simulink model "Digital_Input_Block"  (R2021a)
settings: Solver=FixedStepDiscrete  StartTime=0.0  StopTime=inf  FixedStep=1e-3  RelTol=1e-3  EnableMultiTasking=on
libraries: simulink x9, arduinolib x9
settings Model: SILPILModeSetting=veronly  ExtModeTrigDuration=2  Creator=Admin  LastModifiedBy=Admin
settings OptimizationCC: EnhancedBackFolding=on  PassReuseOutputArgsAs=Individual arguments  ZeroExternalMemoryAtStartup=off  ZeroInternalMemoryAtStartup=off  MaxStackSize=64  OptimizeBlockOrder=speed  DifferentSizesBufferReuse=on  OptimizationCustomize=off  EfficientTunableParamExpr=on
settings DebuggingCC: ParameterTunabilityLossMsg=error
settings HardwareCC: ProdBitPerInt=16  ProdBitPerPointer=16  ProdBitPerSizeT=16  ProdBitPerPtrDiffT=16  ProdLargestAtomicFloat=None  ProdWordSize=8  ProdHWDeviceType=Atmel->AVR
settings SFSimCC: MATLABDynamicMemAlloc=off
settings RTWCC: SystemTargetFile=ert.tlc  HardwareBoard=Arduino Uno  TemplateMakefile=ert_default_tmf  Toolchain=Arduino AVR  BuildConfiguration=Faster Runs
settings CodeAppCC: ForceParamTrailComments=on  IgnoreCustomStorageClasses=off  OperatorAnnotations=on  SimulinkDataObjDesc=on  SFDataObjDesc=on  InsertBlockDesc=on
settings ERTTargetCC: SupportContinuousTime=on  SupportVariableSizeSignals=on  ExtModeStaticAllocSize=250

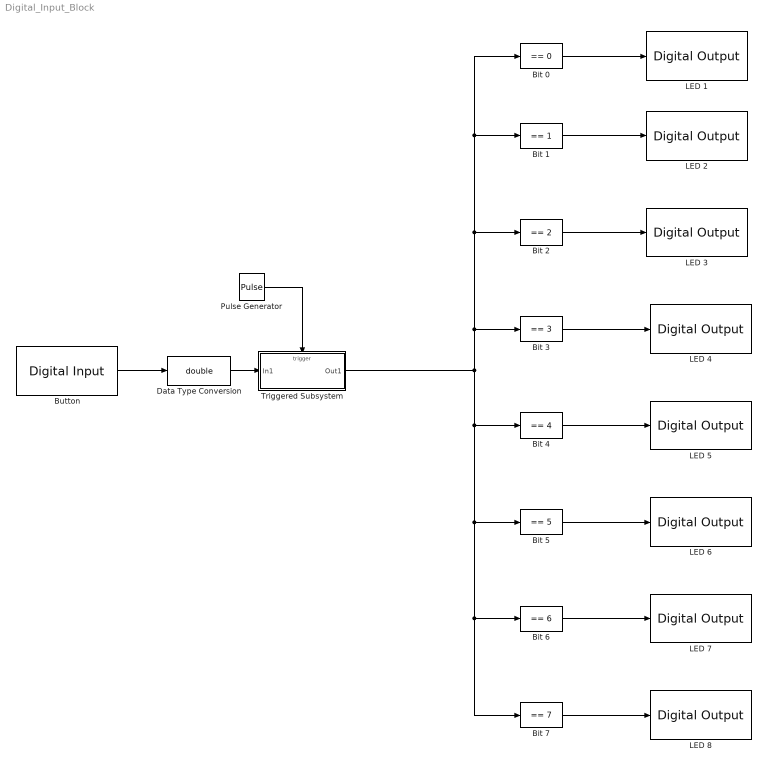
== system Digital_Input_Block ==
  Bit 0 : simulink/Logic and Bit Operations/Compare To Constant  relop===  const=0  OutDataTypeStr=boolean
  Bit 1 : simulink/Logic and Bit Operations/Compare To Constant  relop===  const=1  OutDataTypeStr=boolean
  Bit 2 : simulink/Logic and Bit Operations/Compare To Constant  relop===  const=2  OutDataTypeStr=boolean
  Bit 3 : simulink/Logic and Bit Operations/Compare To Constant  relop===  const=3  OutDataTypeStr=boolean
  Bit 4 : simulink/Logic and Bit Operations/Compare To Constant  relop===  const=4  OutDataTypeStr=boolean
  Bit 5 : simulink/Logic and Bit Operations/Compare To Constant  relop===  const=5  OutDataTypeStr=boolean
  Bit 6 : simulink/Logic and Bit Operations/Compare To Constant  relop===  const=6  OutDataTypeStr=boolean
  Bit 7 : simulink/Logic and Bit Operations/Compare To Constant  relop===  const=7  OutDataTypeStr=boolean
  Button : arduinolib/Digital Input  pinNumber=2  mode=Input Pullup  Direction=input  SampleTime=1e-3  blockPlatform=arduino
  Data Type Conversion : DataTypeConversion  OutDataTypeStr=double
  LED 1 : arduinolib/Digital Output  pinNumber=10  Direction=output  blockPlatform=arduino
  LED 2 : arduinolib/Digital Output  pinNumber=9  Direction=output  blockPlatform=arduino
  LED 3 : arduinolib/Digital Output  pinNumber=8  Direction=output  blockPlatform=arduino
  LED 4 : arduinolib/Digital Output  pinNumber=7  Direction=output  blockPlatform=arduino
  LED 5 : arduinolib/Digital Output  pinNumber=6  Direction=output  blockPlatform=arduino
  LED 6 : arduinolib/Digital Output  pinNumber=5  Direction=output  blockPlatform=arduino
  LED 7 : arduinolib/Digital Output  pinNumber=4  Direction=output  blockPlatform=arduino
  LED 8 : arduinolib/Digital Output  pinNumber=3  Direction=output  blockPlatform=arduino
  Pulse Generator : DiscretePulseGenerator  Period=500  PulseWidth=250  SampleTime=1e-3
  "Triggered Subsystem " : Subsystem  TreatAsAtomicUnit=on
  wires:
  Bit 0/1 -> LED 1/1
  Bit 1/1 -> LED 2/1
  "Triggered Subsystem "/1(Out1) -> Bit 6/1, Bit 7/1, Bit 5/1, Bit 4/1, Bit 0/1, Bit 1/1, Bit 2/1, Bit 3/1
  Bit 7/1 -> LED 8/1
  Bit 6/1 -> LED 7/1
  Bit 5/1 -> LED 6/1
  Bit 4/1 -> LED 5/1
  Bit 3/1 -> LED 4/1
  Bit 2/1 -> LED 3/1
  Button/1 -> Data Type Conversion/1
  Pulse Generator/1 -> "Triggered Subsystem "/Trigger
  Data Type Conversion/1 -> "Triggered Subsystem "/1(In1)

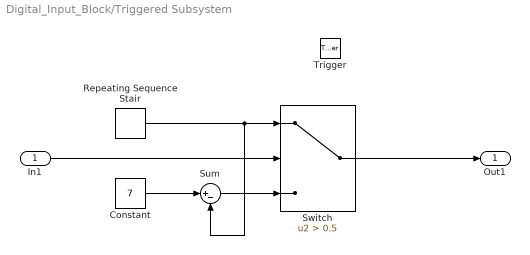
== system Digital_Input_Block/Triggered Subsystem  ==
  In1 : Inport
  Trigger : TriggerPort  VariantControl=(inherit)
  Constant : Constant  Value=7
  Repeating Sequence Stair : simulink/Sources/Repeating Sequence Stair  OutValues=[0 1 2 3 4 5 6 7]  tsamp=-1  OutMin=[]  OutMax=[]  OutDataTypeStr=double  OutputDataTypeScalingMode=double  OutDataType=fixdt(0,8)  ConRadixGroup=Best Precision: Vector-wise  OutScaling=2^-12
  Sum : Sum  Inputs=|+-  AccumDataTypeStr=double
  Switch : Switch  Criteria=u2 > Threshold  Threshold=0.5
  Out1 : Outport
  wires:
  In1/1 -> Switch/2
  Repeating Sequence Stair/1 -> Sum/2, Switch/1
  Switch/1 -> Out1/1
  Constant/1 -> Sum/1
  Sum/1 -> Switch/3
